simulink model "EV_TMS_MODEL"  (R2024a)
settings: Solver=VariableStepAuto  StartTime=0.0  StopTime=1000  RelTol=1e-3
values from neighbouring files (symbols this model uses):
  air_density = 1.225    [model_script.m]
  battery_C1_LUT = [1913.6 12447 30609 ... (first row only)    [model_script.m]
  battery_capacity_LUT = [280.081 276.25 276.392]    [model_script.m]
  battery_cell_cp = 795    [model_script.m]
  battery_cell_mass = 2.5    [model_script.m]
  battery_Em_LUT = [3.4966 3.5057 3.5148 ... (first row only)    [model_script.m]
  battery_N_cells = 20    [model_script.m]
  battery_Qe_init = 0    [model_script.m]
  battery_R0_LUT = [0.0117 0.0085 0.009 ... (first row only)    [model_script.m]
  battery_R1_LUT = [0.0109 0.0029 0.0013 ... (first row only)    [model_script.m]
  battery_SOC_LUT = [0; 0.1; 0.25; 0.5; 0.75; 0.9; 1]    [model_script.m]
  battery_T_init = -10    [model_script.m]
  battery_temperature_LUT = [-10 0 5 20 40]    [model_script.m]
  cabin_doors_conductivity = 0.2    [model_script.m]
  cabin_glass_conductivity = 1    [model_script.m]
  cabin_roof_conductivity = 0.2    [model_script.m]
  cabin_T_init = -10    [model_script.m]
  coolant_channel_D = 0.0092    [model_script.m]
  coolant_pipe_D = 0.02    [model_script.m]
  coolant_T_init = 30    [model_script.m]
  coolant_tank_volume = 5    [model_script.m]
  CoolingPower_kW = 3    [model_script.m]
  duct_W = 0.2    [model_script.m]
  evap_superheat_temp = 5    [model_script.m]
  pump_speed_max = 3000    [model_script.m]
  refrigerant_massflowrate = CoolingPower_kW/(evap_outlet_enthalpy-evap_inlet_enthalpy)    (= 0.0184049079755)    [model_script.m]
  RPM_Compressor_nominal = 1000    [model_script.m]
  RPM_CondFan = 3000    [model_script.m]
  RPM_EvapFan = 3000    [model_script.m]
  T_set = 20    [model_script.m]
  tube_D = 0.01    [model_script.m]
  VolFlowrate_CondenserFan = condenser_air_massflowrate/air_density    (= 0.408163265306)    [model_script.m]
  VolFlowRate_CoolantRadiatorFan = 0.5    [model_script.m]
  VolFlowRate_EvapFan = evap_air_massflowrate/air_density    (= 0.487359122754)    [model_script.m]
undefined symbols (not defined in the file or in its folder): bulb, inlet
libraries: fl_lib x238, nesl_utility x75, SimscapeFluids_lib x25, LiBatteryElements_lib x16, simulink_extras x9, slpidlib x3, autolibshared x1, SignalEditorBlockLib x1
(part 2 of 7)

== system EV_TMS_MODEL/S4 ==
  Absolute Reference (2P) : fl_lib/Two-Phase Fluid/Elements/Absolute Reference (2P)
  PS-Simulink Converter : nesl_utility/PS-Simulink Converter  PhysicalDomain=network_engine_domain  SubClassName=ps_output  LeftPortType=input  RightPortType=output  PseudoPeriodic=off  Frequencies=[]  VectorFormat=inherit  Unit=kJ/kg  AffineConversion=off
  PS-Simulink Converter1 : nesl_utility/PS-Simulink Converter  PhysicalDomain=network_engine_domain  SubClassName=ps_output  LeftPortType=input  RightPortType=output  PseudoPeriodic=off  Frequencies=[]  VectorFormat=inherit  Unit=MPa  AffineConversion=off
  Pressure & Internal Energy Sensor (2P) : fl_lib/Two-Phase Fluid/Sensors/Pressure, Temperature & Internal Energy Sensor (2P)  reference=foundation.enum.MeasurementReference.difference  pressure=true  pressure_spec=foundation.enum.PressureMeasementSpec.Absolute  temperature=false  internal_energy=true
      settings: InternalSimscapePortConfiguration="{\"Bottom\":[{\"id\":\"U\",\"label\":\"U\",\"type\":\"output\"}],\"Left\":[{\"id\":\"A\",\"label\":\"A\",\"type\":\"foundation.two_phase_fluid.two_phase_fluid\"}],\"Right\":[{\"id\":\"B\",\"label\":\"B\",\"type\":\"foundation.two_phase_fluid.two_phase_fluid\"},{\"id\":\"P\",\"label\":\"P\",\"type\":\"output\"}],\"Top\":[]}"
  Saturation Properties Sensor (2P) : fl_lib/Two-Phase Fluid/Sensors/Saturation Properties Sensor (2P)  temperature_measure=true  pressure_measure=simscape.enum.onoff.off  pressure_check=simscape.enum.assert.action.error  energy_measure=foundation.enum.EnergyMeasurement.SaturatedEnthalpy  density_measure=foundation.enum.DensityMeasurement.Off
      settings: InternalSimscapePortConfiguration="{\"Bottom\":[],\"Left\":[{\"id\":\"A\",\"label\":\"A\",\"type\":\"foundation.two_phase_fluid.two_phase_fluid\"}],\"Right\":[{\"id\":\"T_sat_liq\",\"label\":\"TL\",\"type\":\"output\"},{\"id\":\"T_sat_vap\",\"label\":\"TV\",\"type\":\"output\"}],\"Top\":[{\"id\":\"h_sat_liq\",\"label\":\"HL\",\"type\":\"output\"},{\"id\":\"h_sat_vap\",\"label\":\"HV\",\"type\":\"output\"}]}"
  Thermodynamic Properties Sensor (2P) : fl_lib/Two-Phase Fluid/Sensors/Thermodynamic Properties Sensor (2P)  temperature=true  enthalpy=true  density=false  specific_volume=true  entropy=true
      settings: InternalSimscapePortConfiguration="{\"Bottom\":[{\"id\":\"V\",\"label\":\"v\",\"type\":\"output\"},{\"id\":\"S\",\"label\":\"s\",\"type\":\"output\"}],\"Left\":[{\"id\":\"A\",\"label\":\"A\",\"type\":\"foundation.two_phase_fluid.two_phase_fluid\"}],\"Right\":[{\"id\":\"T\",\"label\":\"T\",\"type\":\"output\"},{\"id\":\"H\",\"label\":\"h\",\"type\":\"output\"}],\"Top\":[]}"
  A : PMIOPort  Side=Left
  tag scope: h4=global, p4=global
  wires:
  PS-Simulink Converter/1 -> [h4]
  PS-Simulink Converter1/1 -> [p4]
  connections:
  Pressure & Internal Energy Sensor (2P)/LConn1 -- Saturation Properties Sensor (2P)/LConn1 -- Thermodynamic Properties Sensor (2P)/LConn1 -- A/RConn1
  Absolute Reference (2P)/LConn1 -- Pressure & Internal Energy Sensor (2P)/RConn1
  PS-Simulink Converter/LConn1 -- Thermodynamic Properties Sensor (2P)/RConn2
  PS-Simulink Converter1/LConn1 -- Pressure & Internal Energy Sensor (2P)/RConn2

== system EV_TMS_MODEL/S5 ==
  Absolute Reference (2P) : fl_lib/Two-Phase Fluid/Elements/Absolute Reference (2P)
  PS-Simulink Converter : nesl_utility/PS-Simulink Converter  PhysicalDomain=network_engine_domain  SubClassName=ps_output  LeftPortType=input  RightPortType=output  PseudoPeriodic=off  Frequencies=[]  VectorFormat=inherit  Unit=kJ/kg  AffineConversion=off
  PS-Simulink Converter1 : nesl_utility/PS-Simulink Converter  PhysicalDomain=network_engine_domain  SubClassName=ps_output  LeftPortType=input  RightPortType=output  PseudoPeriodic=off  Frequencies=[]  VectorFormat=inherit  Unit=MPa  AffineConversion=off
  Pressure & Internal Energy Sensor (2P) : fl_lib/Two-Phase Fluid/Sensors/Pressure, Temperature & Internal Energy Sensor (2P)  reference=foundation.enum.MeasurementReference.difference  pressure=true  pressure_spec=foundation.enum.PressureMeasementSpec.Absolute  temperature=false  internal_energy=true
      settings: InternalSimscapePortConfiguration="{\"Bottom\":[{\"id\":\"U\",\"label\":\"U\",\"type\":\"output\"}],\"Left\":[{\"id\":\"A\",\"label\":\"A\",\"type\":\"foundation.two_phase_fluid.two_phase_fluid\"}],\"Right\":[{\"id\":\"B\",\"label\":\"B\",\"type\":\"foundation.two_phase_fluid.two_phase_fluid\"},{\"id\":\"P\",\"label\":\"P\",\"type\":\"output\"}],\"Top\":[]}"
  Saturation Properties Sensor (2P) : fl_lib/Two-Phase Fluid/Sensors/Saturation Properties Sensor (2P)  temperature_measure=true  pressure_measure=simscape.enum.onoff.off  pressure_check=simscape.enum.assert.action.error  energy_measure=foundation.enum.EnergyMeasurement.SaturatedEnthalpy  density_measure=foundation.enum.DensityMeasurement.Off
      settings: InternalSimscapePortConfiguration="{\"Bottom\":[],\"Left\":[{\"id\":\"A\",\"label\":\"A\",\"type\":\"foundation.two_phase_fluid.two_phase_fluid\"}],\"Right\":[{\"id\":\"T_sat_liq\",\"label\":\"TL\",\"type\":\"output\"},{\"id\":\"T_sat_vap\",\"label\":\"TV\",\"type\":\"output\"}],\"Top\":[{\"id\":\"h_sat_liq\",\"label\":\"HL\",\"type\":\"output\"},{\"id\":\"h_sat_vap\",\"label\":\"HV\",\"type\":\"output\"}]}"
  Thermodynamic Properties Sensor (2P) : fl_lib/Two-Phase Fluid/Sensors/Thermodynamic Properties Sensor (2P)  temperature=true  enthalpy=true  density=false  specific_volume=true  entropy=true
      settings: InternalSimscapePortConfiguration="{\"Bottom\":[{\"id\":\"V\",\"label\":\"v\",\"type\":\"output\"},{\"id\":\"S\",\"label\":\"s\",\"type\":\"output\"}],\"Left\":[{\"id\":\"A\",\"label\":\"A\",\"type\":\"foundation.two_phase_fluid.two_phase_fluid\"}],\"Right\":[{\"id\":\"T\",\"label\":\"T\",\"type\":\"output\"},{\"id\":\"H\",\"label\":\"h\",\"type\":\"output\"}],\"Top\":[]}"
  A : PMIOPort  Side=Left
  tag scope: h5=global, p5=global
  wires:
  PS-Simulink Converter/1 -> [h5]
  PS-Simulink Converter1/1 -> [p5]
  connections:
  Pressure & Internal Energy Sensor (2P)/LConn1 -- Saturation Properties Sensor (2P)/LConn1 -- Thermodynamic Properties Sensor (2P)/LConn1 -- A/RConn1
  Absolute Reference (2P)/LConn1 -- Pressure & Internal Energy Sensor (2P)/RConn1
  PS-Simulink Converter/LConn1 -- Thermodynamic Properties Sensor (2P)/RConn2
  PS-Simulink Converter1/LConn1 -- Pressure & Internal Energy Sensor (2P)/RConn2

== system EV_TMS_MODEL/Subsystem ==
  Drive Cycle Source : autolibshared/Drive Cycle Source  cycleVar=UDDS  fileVar=cycleFTP75.mat  tfinal="1369  seconds"  cycleRepeat=off  outAccPort=off  outGearPort=off  gearList=No gear data  t_wot1=5  xdot_woto=0  xdot_wot1=30  t_wot2=20  xdot_wot2=0  t_wotend=30  srcUnit=m/s  outUnit=m/s  srcAccUnit=m/s/s  outAccUnit=m/s^2  dt=0  aMode=2  faultOption=off  velBnd=2  velBndUnit=mph  inUnit=m/s  timeBnd=1  failOption=off  stopSim=off  maxFaultCnt=10  maxFaultTime=2  maxTotFaultTime=15  traceOption=off  dtTrace=1  traceWindow=10  lastDCname=UDDS  lastOutUnit=mph  lastDT=0  lastTB=1  lastSB=2  forceCalcBound=off
      settings: LibrarySourceBlock=vdynlib/Vehicle Scenarios/Drive Cycle and Maneuvers/Drive Cycle Source
  Goto : Goto  Commented=on  GotoTag=I_battery  TagVisibility=global
  Goto1 : Goto  Commented=on  GotoTag=Q_inverter  TagVisibility=global
  Goto11 : Goto  Commented=on  GotoTag=Q_charger  TagVisibility=global
  Goto3 : Goto  Commented=on  GotoTag=Q_motor  TagVisibility=global
  Goto7 : Goto  Commented=on  GotoTag=v_vehicle  TagVisibility=global
  Power Demand : Subsystem  Commented=on
  Power Demand1 : Subsystem
  Signal Editor : SignalEditorBlockLib/Signal Editor  Commented=on  FileName=EVBatteryCoolingSystem.mat  ActiveScenario=FTP_75_Drive_Cycle  ActiveSignal=Speed  IsBus=off  OutputBusObjectStr=Bus: BusObject  SampleTime=0  Interpolate=off  ZeroCross=off  OutputAfterFinalValue=Setting to zero  Unit=inherit  PreserveSignalName=on  ApplySigPropsToAllScenarios=on  ApplySigPropsToAllSignals=off
  tag scope: I_battery=global, Q_charger=global, Q_inverter=global, Q_motor=global, v_vehicle=global
  wires:
  Power Demand/4(Q_charger) -> Goto11/1
  Power Demand/2(Q_inverter) -> Goto1/1
  Power Demand/1(I_battery) -> Goto/1
  Power Demand/3(Q_motor) -> Goto3/1
  Signal Editor/1 -> Power Demand/1(speed), Goto7/1
  Signal Editor/2 -> Power Demand/2(In2)
  Power Demand1/2(Q_inverter) -> [Q_inverter]
  Power Demand1/3(Q_motor) -> [Q_motor]
  Power Demand1/1(I_battery) -> [I_battery]
  Power Demand1/4(Q_charger) -> [Q_charger]
  Drive Cycle Source/1 -> [v_vehicle], Power Demand1/1(speed)

== system EV_TMS_MODEL/Subsystem1 ==
  Sum : Sum  Inputs=|+++++
  Out1 : Outport
  wires:
  [Q_chiller] -> Sum/3  "ChillerHeat"
  [Q_coolant_radiator] -> Sum/5  "CoolantRadiatorHeat"
  [Q_cond] -> Sum/1  "CondenserHeat"
  Sum/1 -> Out1/1
  [Q_cabin] -> Sum/4  "CabinHeatExchangeToExterior"
  [Q_evap] -> Sum/2  "EvaporatorHeat"

== system EV_TMS_MODEL/Subsystem2 ==
  Sum : Sum  Inputs=|+++++
  Out1 : Outport
  wires:
  Sum/1 -> Out1/1
  [Pwr_CoolantPump] -> Sum/4  "Pwr_CoolantPump"
  [Pwr_CoolantRadiatorFan] -> Sum/5  "Pwr_CoolantRadiatorFan"
  [Pwr_Compressor] -> Sum/1  "Pwr_Compressor"
  [Pwr_CondenserFan] -> Sum/2  "Pwr_CondenserFan"
  [Pwr_BlowerFan] -> Sum/3  "Pwr_BlowerFan"

== system EV_TMS_MODEL/TXV1 ==
  note: The bulb of the TXV contains a temperature-sensitive material (such as a refrigerant) that expands or contracts based on the temperature it is exposed to. This expansion or contraction of the bulb material controls the opening and closing of the TXV valve, regulating the flow of refrigerant into the evaporator coil. The bulb temperature is typically measured at the outlet of the evaporator coil. The bulb of the TXV is attached to the suction line of the refrigeration system at the outlet of the evaporator, the line which is connected to the compressor. This placement allows the bulb to sense the temperature of the refrigerant vapor leaving the evaporator.
      | By measuring the temperature at the outlet of the evaporator, the TXV can maintain a consistent superheat level, ensuring optimal evaporator performance and preventing issues such as flooding or starving of the evaporator coil. The superheat level is the difference between the measured bulb temperature and the refrigerant saturation temperature at the evaporator outlet.
  Simscape Bus : SimscapeBus  HierarchyStrings=bulb;inlet
  Thermostatic Expansion Valve : SimscapeFluids_lib/Two-Phase Fluid/Valves & Orifices/Flow Control Valves/Thermostatic Expansion Valve (2P)  valve_parameterization=fluids.two_phase_fluid.valves_orifices.flow_control_valves.enum.ThermostaticExpansionValveParameterization.Nominal  capacity_spec=fluids.two_phase_fluid.valves_orifices.flow_control_valves.enum.ThermostaticExpansionValveCapacitySpec.MassFlowRate  Q_nominal=0.5*CoolingPower_kW kW  Q_max=0.5*CoolingPower_kW* 1.5 kW  mdot_nominal=refrigerant_massflowrate kg/s  mdot_max=1.5*refrigerant_massflowrate kg/s  pressure_spec=fluids.two_phase_fluid.valves_orifices.flow_control_valves.enum.ThermostaticExpansionValvePressureSpec.SaturationTemperature  p_cond_nominal=1.5 MPa  p_evap_nominal=0.5 MPa  T_cond_nominal=nominal_condens_temp degC  T_evap_nominal=nominal_evap_temp degC  delta_T_sub=condenser_subcooling_temp deltaK  delta_T_nominal=evap_superheat_temp deltaK  delta_T_static=0.5*evap_superheat_temp deltaK  mop=fluids.two_phase_fluid.valves_orifices.flow_control_valves.enum.ThermostaticExpansionValveMOP.Off  p_mop=0.5 MPa  T_mop=288.15 K  T_evap_out_TLU1=0 : 10 : 40 degC  p_bulb_TLU1=0.3 : 0.1 : 0.7 MPa  lift_TLU2=0 : 0.15 : 0.6 mm  p_evap_TLU2=0.3 : -0.05 : 0.1 MPa  lift_TLU3=0 : 0.15 : 0.6 mm  mdot_TLU3=0 : 0.015 : 0.06 kg/s  p_cond_ref=2 MPa  p_evap_ref=0.2 MPa  T_evap_out_ref=0 degC  delta_T_sub_ref=5 deltaK  pressure_equalization=fluids.two_phase_fluid.valves_orifices.flow_control_valves.enum.ThermostaticExpansionValveEqualization.External  bulb_dynamics=simscape.enum.onoff.off  tau_bulb=20 s  leakage_fraction=1e-6  smoothing_factor=0.5  B_lam=0.999  tau_x=0.1 s  area=pi*tube_D^2/4 m^2
      settings: InternalSimscapePortConfiguration="{\"Bottom\":[],\"Left\":[{\"id\":\"A\",\"label\":\"A\",\"type\":\"foundation.two_phase_fluid.two_phase_fluid\"}],\"Right\":[{\"id\":\"B\",\"label\":\"B\",\"type\":\"foundation.two_phase_fluid.two_phase_fluid\"}],\"Top\":[{\"id\":\"S\",\"label\":\"S\",\"type\":\"foundation.two_phase_fluid.two_phase_fluid\"},{\"id\":\"E\",\"label\":\"E\",\"type\":\"foundation.two_phase_fluid.two_phase_fluid\"}]}"
  B : PMIOPort  Side=Left
  A : PMIOPort  Port=2  Side=Right
  connections:
  B/RConn1 -- Simscape Bus/RConn1
  Thermostatic Expansion Valve/RConn1 -- Simscape Bus/LConn2
  Simscape Bus/LConn1 -- Thermostatic Expansion Valve/LConn2 -- Thermostatic Expansion Valve/LConn3
  Thermostatic Expansion Valve/LConn1 -- A/RConn1

== system EV_TMS_MODEL/TXV2 ==
  note: The bulb of the TXV contains a temperature-sensitive material (such as a refrigerant) that expands or contracts based on the temperature it is exposed to. This expansion or contraction of the bulb material controls the opening and closing of the TXV valve, regulating the flow of refrigerant into the evaporator coil. The bulb temperature is typically measured at the outlet of the evaporator coil. The bulb of the TXV is attached to the suction line of the refrigeration system at the outlet of the evaporator, the line which is connected to the compressor. This placement allows the bulb to sense the temperature of the refrigerant vapor leaving the evaporator.
      | By measuring the temperature at the outlet of the evaporator, the TXV can maintain a consistent superheat level, ensuring optimal evaporator performance and preventing issues such as flooding or starving of the evaporator coil. The superheat level is the difference between the measured bulb temperature and the refrigerant saturation temperature at the evaporator outlet.
  Chiller Expansion Valve : SimscapeFluids_lib/Two-Phase Fluid/Valves & Orifices/Flow Control Valves/Thermostatic Expansion Valve (2P)  valve_parameterization=fluids.two_phase_fluid.valves_orifices.flow_control_valves.enum.ThermostaticExpansionValveParameterization.Nominal  capacity_spec=fluids.two_phase_fluid.valves_orifices.flow_control_valves.enum.ThermostaticExpansionValveCapacitySpec.MassFlowRate  Q_nominal=CoolingPower_kW kW  Q_max=CoolingPower_kW* 1.5 kW  mdot_nominal=refrigerant_massflowrate kg/s  mdot_max=1.5*refrigerant_massflowrate kg/s  pressure_spec=fluids.two_phase_fluid.valves_orifices.flow_control_valves.enum.ThermostaticExpansionValvePressureSpec.SaturationTemperature  p_cond_nominal=1.5 MPa  p_evap_nominal=0.3 MPa  T_cond_nominal=nominal_condens_temp degC  T_evap_nominal=nominal_evap_temp degC  delta_T_sub=condenser_subcooling_temp deltaK  delta_T_nominal=evap_superheat_temp deltaK  delta_T_static=0.5*evap_superheat_temp deltaK  mop=fluids.two_phase_fluid.valves_orifices.flow_control_valves.enum.ThermostaticExpansionValveMOP.Off  p_mop=0.5 MPa  T_mop=288.15 K  T_evap_out_TLU1=0 : 10 : 40 degC  p_bulb_TLU1=0.3 : 0.1 : 0.7 MPa  lift_TLU2=0 : 0.15 : 0.6 mm  p_evap_TLU2=0.3 : -0.05 : 0.1 MPa  lift_TLU3=0 : 0.15 : 0.6 mm  mdot_TLU3=[1e-7, 0.015 : 0.015 : 0.06] kg/s  p_cond_ref=2 MPa  p_evap_ref=0.3 MPa  T_evap_out_ref=0 degC  delta_T_sub_ref=5 deltaK  pressure_equalization=fluids.two_phase_fluid.valves_orifices.flow_control_valves.enum.ThermostaticExpansionValveEqualization.External  bulb_dynamics=false  tau_bulb=20 s  leakage_fraction=1e-6  smoothing_factor=0.5  B_lam=0.999  tau_x=1 s  area=pi*tube_D^2/4 m^2
      settings: InternalSimscapePortConfiguration="{\"Bottom\":[],\"Left\":[{\"id\":\"A\",\"label\":\"A\",\"type\":\"foundation.two_phase_fluid.two_phase_fluid\"}],\"Right\":[{\"id\":\"B\",\"label\":\"B\",\"type\":\"foundation.two_phase_fluid.two_phase_fluid\"}],\"Top\":[{\"id\":\"S\",\"label\":\"S\",\"type\":\"foundation.two_phase_fluid.two_phase_fluid\"},{\"id\":\"E\",\"label\":\"E\",\"type\":\"foundation.two_phase_fluid.two_phase_fluid\"}]}"
  Simscape Bus : SimscapeBus  HierarchyStrings=bulb;inlet
  B : PMIOPort  Side=Left
  A : PMIOPort  Port=2  Side=Right
  connections:
  Simscape Bus/RConn1 -- B/RConn1
  Simscape Bus/LConn1 -- Chiller Expansion Valve/LConn2 -- Chiller Expansion Valve/LConn3
  Simscape Bus/LConn2 -- Chiller Expansion Valve/RConn1
  A/RConn1 -- Chiller Expansion Valve/LConn1

== system EV_TMS_MODEL/Cabin/Cabin ==
  Cabin and Occupants Model : Subsystem  Tag=PublishSubsystem
      settings: PortSchema="{\"entries\":[{\"content\":{\"sides\":[{\"content\":{},\"type\":\"ConnectorPlacement.EquallySpacedRectSide\",\"uuid\":\"e1f7673a-ae09-4e38-a748-d03f3a89f634\"},{\"content\":{\"connectorIds\":[\"RConn1\"],\"side\":\"RIGHT\"},\"type\":\"ConnectorPlacement.EquallySpacedRectSide\",\"uuid\":\"e2c59df4-5a81-4f6b-ab06-631ef800c0b1\"},{\"content\":{\"connectorIds\":[\"LConn1\"],\"side\":\"TOP\"},\"type\":\"ConnectorPlacement.EquallySpacedRectSide\",\"uuid\":\"19dd88a8-04e0-4296-a227-9de66059cdf8\"}]},\"type\":\"ConnectorPlacement.EquallySpacedConnector\",\"uuid\":\"cfca4f7e-9c0e-462b-910e-b09b0fceba6e\"}],\"packageUris\":[\"http://schema.mathworks.com/mf0/Connector/R2020b\"],\"version\":\"1.0\"}"
      settings: AttributesFormatString=|
      | Length= %<coolingBox_L>
      | Width= %<coolingBox_W>
      | Height= %<coolingBox_H>
      | Initial Temp= %<T_cabin_init_degC>
  Evaporator A : PMIOPort  Side=Left
  Evaporator B : PMIOPort  Port=2  Side=Left
  connections:
  Evaporator B/RConn1 -- Cabin and Occupants Model/LConn1
  Evaporator A/RConn1 -- Cabin and Occupants Model/RConn1

== system EV_TMS_MODEL/Chiller/Chiller ==
  note: Heat exchanger (system-level model) that lets the refrigerant absorb heat from the coolant.This way the coolant (water glycol) from the battery is cooled and heats the refrigerant (R410a)
  note: This is a model of a chiller that uses two-phase refrigeration circuit to cool a thermal liquid network. The thermal liquid network uses a water-based coolant fluid and the model can be expanded to model cooling of a BEV or HEV battery, DC/DC converter, inverter, electric motors, etc.
  Chiller (System-Level) : SimscapeFluids_lib/Heat Exchangers/Two-Phase Fluid - Thermal Liquid/System-Level Condenser Evaporator (2P-TL)  flow_arrangement=fluids.heat_exchangers.enum.SystemLevelFlowArrangement2PTL.Cross  wall_thermal_mass=false  mass_wall=1 kg  cp_wall=490 J/(K*kg)  nominal_init_wall=true  T_wall_init=293.15 K  area_A1=pi*tube_D^2/4 m^2  area_B1=pi*tube_D^2/4 m^2  area_A2=pi*tube_D^2/4 m^2  area_B2=pi*tube_D^2/4 m^2  operating_condition_2P=fluids.heat_exchangers.enum.SystemLevelOperatingCondition2PTL.Evaporator  mdot_nominal_2P=0.5*refrigerant_massflowrate kg/s  delta_p_nominal_2P=0.01 MPa  pressure_spec_cond_2P=fluids.heat_exchangers.enum.SystemLevelPressureSpecCondenser2P.InletPressure  pressure_spec_evap_2P=fluids.heat_exchangers.enum.SystemLevelPressureSpecEvaporator2P.EvaporatingTemperature  p_in_nominal_2P=1 MPa  T_cond_nominal_2P=313.15 K  T_evap_nominal_2P=nominal_evap_temp degC  inlet_spec_2P=fluids.heat_exchangers.enum.SystemLevelInletSpec2P.Temperature  T_in_nominal_2P=-10 degC  h_in_nominal_2P=evap_inlet_enthalpy kJ/kg  x_in_nominal_2P=1  capacity_spec_2P=fluids.heat_exchangers.enum.SystemLevelCapacitySpec.HeatTransfer  Q_nominal=0.1 kW  outlet_spec_cond_2P=fluids.heat_exchangers.enum.SystemLevelOutletSpecCondenser2P.Enthalpy  outlet_spec_evap_2P=fluids.heat_exchangers.enum.SystemLevelOutletSpecEvaporator2P.Superheating  delta_T_sub_nominal_2P=5 deltaK  delta_T_sup_nominal_2P=evap_superheat_temp deltaK  h_out_nominal_2P=250 kJ/kg  x_out_nominal_2P=0  volume_2P=0.001 m^3  nominal_init_2P=false  energy_spec_2P=foundation.enum.energy_spec.temperature  p_init_2P=evap_inlet_p MPa  T_init_2P=9 degC  x_init_2P=0.5  alpha_init_2P=0.5  h_init_2P=evap_inlet_enthalpy kJ/kg  u_init_2P=1500 kJ/kg  mdot_nominal_TL=pump_nominal_massflowrate kg/s  delta_p_nominal_TL=0.01 MPa  p_in_nominal_TL=coolant_p_init MPa  T_in_nominal_TL=coolant_T_init degC  volume_TL=0.001 m^3  nominal_init_TL=true  p_init_TL=0.101325 MPa  T_init_TL=293.15 K  a_liq_2P=0.023  a_mix_2P=0.005  a_vap_2P=0.023  b_2P=0.8  c_2P=0.33  a_TL=0.023  b_TL=0.8  c_TL=0.33
      settings: InternalSimscapePortConfiguration="{\"Bottom\":[],\"Left\":[{\"id\":\"A1\",\"label\":\"A1\",\"type\":\"foundation.two_phase_fluid.two_phase_fluid\"},{\"id\":\"B1\",\"label\":\"B1\",\"type\":\"foundation.two_phase_fluid.two_phase_fluid\"}],\"Right\":[{\"id\":\"A2\",\"label\":\"A2\",\"type\":\"foundation.thermal_liquid.thermal_liquid\"},{\"id\":\"B2\",\"label\":\"B2\",\"type\":\"foundation.thermal_liquid.thermal_liquid\"}],\"Top\":[{\"id\":\"Q1\",\"label\":\"Q1\",\"type\":\"output\"},{\"id\":\"Q2\",\"label\":\"Q2\",\"type\":\"output\"}]}"
  PS-Simulink Converter1 : nesl_utility/PS-Simulink Converter  PhysicalDomain=network_engine_domain  SubClassName=ps_output  LeftPortType=input  RightPortType=output  PseudoPeriodic=off  Frequencies=[]  VectorFormat=inherit  Unit=kW  AffineConversion=off
  Simscape Bus : SimscapeBus  HierarchyStrings=bulb;inlet
  To Compressor : PMIOPort  Side=Left
  C : PMIOPort  Port=2  Side=Left
  D : PMIOPort  Port=3  Side=Left
  To TXV : PMIOPort  Port=4  Side=Right
  Heat flow rate [kW] : Outport
  wires:
  PS-Simulink Converter1/1 -> Heat flow rate [kW]/1
  connections:
  To TXV/RConn1 -- Simscape Bus/RConn1
  Simscape Bus/LConn1 -- Chiller (System-Level)/LConn2 -- To Compressor/RConn1
  Simscape Bus/LConn2 -- Chiller (System-Level)/LConn1
  Chiller (System-Level)/RConn1 -- C/RConn1
  Chiller (System-Level)/RConn2 -- D/RConn1
  PS-Simulink Converter1/LConn1 -- Chiller (System-Level)/LConn3

== system EV_TMS_MODEL/Compressor/Compressor ==
  Compressor On/Off : Inport
  Compressor : Subsystem  Variant=on  VariantControlMode=label  LabelModeActiveChoice=Compressor_detailed
  Evap Outlet : PMIOPort  Side=Left
  Condenser Inlet : PMIOPort  Port=2  Side=Right
  Power [kW] : Outport
  wires:
  Compressor On/Off/1 -> Compressor/1(Compressor On/Off)
  Compressor/1(Power [kW]) -> Power [kW]/1
  connections:
  Evap Outlet/RConn1 -- Compressor/LConn1
  Condenser Inlet/RConn1 -- Compressor/RConn1

== system EV_TMS_MODEL/Condenser and Fan/Condenser and Fan ==
  Fan On/Off : Inport
  Condenser (System-Level) : SimscapeFluids_lib/Heat Exchangers/Two-Phase Fluid - Moist Air/System-Level Condenser Evaporator (2P-MA)  flow_arrangement=fluids.heat_exchangers.enum.SystemLevelFlowArrangement2PMA.Cross  wall_thermal_mass=simscape.enum.onoff.off  mass_wall=1 kg  cp_wall=490 J/(K*kg)  nominal_init_wall=true  T_wall_init=293.15 K  area_A1=pi*tube_D^2/4 m^2  area_B1=pi*tube_D^2/4 m^2  area_A2=duct_W^2 m^2  area_B2=duct_W^2 m^2  operating_condition_2P=fluids.heat_exchangers.enum.SystemLevelOperatingCondition2PMA.Condenser  mdot_nominal_2P=refrigerant_massflowrate kg/s  delta_p_nominal_2P=0.01 MPa  pressure_spec_cond_2P=fluids.heat_exchangers.enum.SystemLevelPressureSpecCondenser2P.CondensingTemperature  pressure_spec_evap_2P=fluids.heat_exchangers.enum.SystemLevelPressureSpecEvaporator2P.InletPressure  p_in_nominal_2P=1 MPa  T_cond_nominal_2P=nominal_condens_temp degC  T_evap_nominal_2P=243.15 K  inlet_spec_2P=fluids.heat_exchangers.enum.SystemLevelInletSpec2P.Enthalpy  T_in_nominal_2P=condenser_inlet_temp degC  h_in_nominal_2P=460 kJ/kg  x_in_nominal_2P=1  capacity_spec_2P=fluids.heat_exchangers.enum.SystemLevelCapacitySpec.OutletCondition  Q_nominal=0.01 kW  outlet_spec_cond_2P=fluids.heat_exchangers.enum.SystemLevelOutletSpecCondenser2P.Subcooling  outlet_spec_evap_2P=fluids.heat_exchangers.enum.SystemLevelOutletSpecEvaporator2P.Enthalpy  delta_T_sub_nominal_2P=condenser_subcooling_temp deltaK  delta_T_sup_nominal_2P=5 deltaK  h_out_nominal_2P=condenser_inlet_p kJ/kg  x_out_nominal_2P=0  volume_2P=0.001 m^3  nominal_init_2P=true  energy_spec_2P=foundation.enum.energy_spec.enthalpy  p_init_2P=condenser_inlet_p MPa  T_init_2P=refrig_T_init degC  x_init_2P=0.5  alpha_init_2P=0.5  h_init_2P=condenser_inlet_enthalpy kJ/kg  u_init_2P=1500 kJ/kg  mdot_nominal_MA=evap_air_massflowrate kg/s  delta_p_nominal_MA=200 Pa  p_in_nominal_MA=0.101325 MPa  T_in_nominal_MA=T_set degC  inlet_moisture_spec_MA=foundation.enum.moisture_spec.relative_humidity  RH_in_nominal_MA=0.5  x_w_in_nominal_MA=0.01  y_w_in_nominal_MA=0.01  HR_in_nominal_MA=0.01  Tw_in_nominal_MA=287 K  inlet_trace_gas_spec_MA=foundation.enum.trace_gas_spec.mole_fraction  x_g_in_nominal_MA=0.001  y_g_in_nominal_MA=0  volume_MA=0.15 m^3  nominal_init_MA=true  p_init_MA=moist_air_p_init MPa  T_init_MA=moist_air_T_init degC  moisture_spec_MA=foundation.enum.moisture_spec.relative_humidity  RH_init_MA=moist_air_RH_init  x_w_init_MA=0.01  y_w_init_MA=0.01  HR_init_MA=0.01  Tw_init_MA=287 K  trace_gas_spec_MA=foundation.enum.trace_gas_spec.mass_fraction  x_g_init_MA=0.001  y_g_init_MA=0.001  RH_ws_MA=1  a_liq_2P=0.023  a_mix_2P=0.005  a_vap_2P=0.023  b_2P=0.8  c_2P=0.33  a_MA=0.023  b_MA=0.8  c_MA=0.33
      settings: InternalSimscapePortConfiguration="{\"Bottom\":[],\"Left\":[{\"id\":\"A1\",\"label\":\"A1\",\"type\":\"foundation.two_phase_fluid.two_phase_fluid\"},{\"id\":\"B1\",\"label\":\"B1\",\"type\":\"foundation.two_phase_fluid.two_phase_fluid\"}],\"Right\":[{\"id\":\"A2\",\"label\":\"A2\",\"type\":\"foundation.moist_air.moist_air\"},{\"id\":\"B2\",\"label\":\"B2\",\"type\":\"foundation.moist_air.moist_air\"}],\"Top\":[{\"id\":\"Q1\",\"label\":\"Q1\",\"type\":\"output\"},{\"id\":\"Q2\",\"label\":\"Q2\",\"type\":\"output\"},{\"id\":\"W\",\"label\":\"W\",\"type\":\"output\"}]}"
  Fan : Subsystem  Variant=on  VariantControlMode=label  LabelModeActiveChoice=Fan_simple
  PS-Simulink Converter : nesl_utility/PS-Simulink Converter  PhysicalDomain=network_engine_domain  SubClassName=ps_output  LeftPortType=input  RightPortType=output  PseudoPeriodic=off  Frequencies=[]  VectorFormat=inherit  Unit=kW  AffineConversion=off
  Pipe pressure drop : fl_lib/Two-Phase Fluid/Elements/Flow Resistance (2P)  delta_p_nominal=100 Pa  mdot_nominal=refrigerant_massflowrate kg/s  v_nominal=0 m^3/kg  area=pi*tube_D^2/4 m^2  laminar_fraction=1e-3
      settings: InternalSimscapePortConfiguration="{\"Bottom\":[],\"Left\":[{\"id\":\"A\",\"label\":\"A\",\"type\":\"foundation.two_phase_fluid.two_phase_fluid\"}],\"Right\":[{\"id\":\"B\",\"label\":\"B\",\"type\":\"foundation.two_phase_fluid.two_phase_fluid\"}],\"Top\":[]}"
  Air Inlet : PMIOPort  Side=Left
  Air Outlet : PMIOPort  Port=2  Side=Left
  CoolSide_Condenser : PMIOPort  Port=3  Side=Right
  WarmSide_Condenser (from Compressor) : PMIOPort  Port=4  Side=Right
  Heat Power [kW] : Outport
  Fan Power [kW] : Outport  Port=2
  wires:
  Fan On/Off/1 -> Fan/1(Fan On/Off)
  Fan/1(Power [kW]) -> Fan Power [kW]/1
  PS-Simulink Converter/1 -> Heat Power [kW]/1
  connections:
  Air Outlet/RConn1 -- Condenser (System-Level)/RConn2
  Air Inlet/RConn1 -- Fan/RConn1
  Condenser (System-Level)/LConn2 -- CoolSide_Condenser/RConn1
  WarmSide_Condenser (from Compressor)/RConn1 -- Pipe pressure drop/LConn1
  PS-Simulink Converter/LConn1 -- Condenser (System-Level)/LConn4
  Pipe pressure drop/RConn1 -- Condenser (System-Level)/LConn1
  Fan/RConn2 -- Condenser (System-Level)/RConn1

== system EV_TMS_MODEL/Control/Cabin Air Control ==
  note: if the outside temperature is higher then the setpoint temperature turn off the PTC
  T_cabin : Inport
  T_setpoint : Inport  Port=2
  T_env : Inport  Port=3
  T_ptc : Inport  Port=4
  Constant : Constant  Value=0
  PID Controller : slpidlib/PID Controller  Controller=PI  Form=Ideal  TimeDomain=Continuous-time  UseExternalTs=off  SampleTime=-1  IntegratorMethod=Forward Euler  FilterMethod=Forward Euler  ControllerParametersSource=internal  P=1/50  I=1/150  UseKiTs=off  D=0  UseExternalDerivativeSource=off  N=100  UseFilter=on  TunerSelectOption=Transfer Function Based (PID Tuner App)  InitialConditionSource=internal  InitialConditionForIntegrator=0  InitialConditionForFilter=0  DifferentiatorICPrevScaledInput=0  ExternalReset=none  TrackingMode=off  Kt=1  LimitOutput=on  SatLimitsSource=internal  UpperSaturationLimit=1  LowerSaturationLimit=0  LinearizeAsGain=on  AntiWindupMode=back-calculation  Kb=1  LimitIntegrator=off  UpperIntegratorSaturationLimit=inf  LowerIntegratorSaturationLimit=-inf  POutMin=[]  POutMax=[]  IOutMin=[]  IOutMax=[]  DOutMin=[]  DOutMax=[]  NOutMin=[]  NOutMax=[]  SumOutMin=[]  SumOutMax=[]  SaturationOutMin=[]  SaturationOutMax=[]  PParamMin=[]  PParamMax=[]  IParamMin=[]  IParamMax=[]  DParamMin=[]  DParamMax=[]  NParamMin=[]  NParamMax=[]  KbParamMin=[]  KbParamMax=[]  KtParamMin=[]  KtParamMax=[]  KbOutMin=[]  KbOutMax=[]  KtOutMin=[]  KtOutMax=[]  IntegratorOutMin=[]  IntegratorOutMax=[]  FilterOutMin=[]  FilterOutMax=[]  SumI1OutMin=[]  SumI1OutMax=[]  SumI2OutMin=[]  SumI2OutMax=[]  SumI3OutMin=[]  SumI3OutMax=[]  SumI4OutMin=[]  SumI4OutMax=[]  SumDOutMin=[]  SumDOutMax=[]  DifferentiatorOutMin=[]  DifferentiatorOutMax=[]  FilterDiffOutCoefMin=[]  FilterDiffOutCoefMax=[]  ReciprocalOutMin=[]  ReciprocalOutMax=[]  SumDenOutMin=[]  SumDenOutMax=[]  SumNumOutMin=[]  SumNumOutMax=[]  DivideOutMin=[]  DivideOutMax=[]  UdiffTsProdOutMin=[]  UdiffTsProdOutMax=[]  NTsProdOutMin=[]  NTsProdOutMax=[]  UintegralTsProdOutMin=[]  UintegralTsProdOutMax=[]  UngainTsProdOutMin=[]  UngainTsProdOutMax=[]  ClampingZeroOutDataTypeStr=Inherit: Inherit via back propagation  ClampingZeroOutMin=[]  ClampingZeroOutMax=[]  FilterDenConstantOutDataTypeStr=Inherit: Inherit via back propagation  FilterDenConstantOutMin=[]  FilterDenConstantOutMax=[]  PCopyOutDataTypeStr=Inherit: Inherit via back propagation  PCopyOutMin=[]  PCopyOutMax=[]  NCopyOutDataTypeStr=Inherit: Inherit via back propagation  NCopyOutMin=[]  NCopyOutMax=[]  IntegratorContinuousStateAttributes=''  IntegratorStateMustResolveToSignalObject=off  IntegratorRTWStateStorageClass=Auto  FilterContinuousStateAttributes=''  FilterStateMustResolveToSignalObject=off  FilterRTWStateStorageClass=Auto  ParallelPVariant=Passthrough  IdealPVariant=InternalParameters  IVariant=InternalParameters  DVariant=Disabled  IntegratorVariant=Continuous  SatVariant=Enabled  AWVariant=BackCalculation  PCopyVariant=Disabled  TRVariant=Disabled  FdbkBlocksVariant=Forward  IdealPFdbkVariant=Disabled  SatFdbkVariant=Disabled  DerivativeFilterVariant=Disabled  NVariant=Disabled  NCopyVariant=Disabled_SignalSpec  FilterICVariant=Disabled  IntegratorICVariant=InternalICs  ExternalResetVariant=Disabled  TRSumVariant=Passthrough  SumFdbkVariant=Disabled  SumVariant=Sum_PI  TsampFilterVariant=InternalTs  TsampNgainVariant=Passthrough  TsampIntegralVariant=Disabled_SignalSpec  ExternalSaturationOutDataTypeStr=Inherit: Same as second input  DerivativeSourceVariant=Disabled
  Product : Product
  Relay : Relay  OnSwitchValue=45  OffSwitchValue=35  OnOutputValue=0  OffOutputValue=1  ZeroCross=off
  Sign : Signum
  Sum : Sum  Inputs=-+|
  Sum1 : Sum  Inputs=-+|
  Switch : Switch  SaturateOnIntegerOverflow=off  InputSameDT=off
  cmd_blower : Outport
  cmd_ptc : Outport  Port=2
  wires:
  T_setpoint/1 -> Sum1/1, Sum/1
  Sum1/1 -> Switch/2, Sign/1
  Product/1 -> PID Controller/1
  PID Controller/1 -> cmd_blower/1
  T_env/1 -> Sum1/2
  Sum/1 -> Product/1
  Sign/1 -> Product/2
  Constant/1 -> Switch/1
  Switch/1 -> cmd_ptc/1
  Relay/1 -> Switch/3
  T_ptc/1 -> Relay/1
  T_cabin/1 -> Sum/2

== system EV_TMS_MODEL/Control/Coolant Loop Control ==
  T_env : Inport
  T_coolant_battery_in : Inport  Port=2
  T_motor : Inport  Port=3
  T_battery : Inport  Port=4
  Battery Heater : Subsystem
  Battery Pump : Subsystem
  Motor Pump : Subsystem
  cmd_heater : Outport
  cmd_motor_pump : Outport  Port=2
  cmd_battery_pump : Outport  Port=3
  wires:
  Motor Pump/1(cmd_motor_pump) -> Battery Pump/1(cmd_motor_pump), cmd_motor_pump/1
  T_env/1 -> Battery Heater/1(T_env)
  T_coolant_battery_in/1 -> Battery Heater/2(T_coolant_battery_in)
  T_motor/1 -> Motor Pump/1(T_motor)
  Battery Heater/1(cmd_heater) -> cmd_heater/1
  Battery Pump/1(cmd_battery_pump) -> cmd_battery_pump/1
  T_battery/1 -> Battery Pump/2(T_battery)

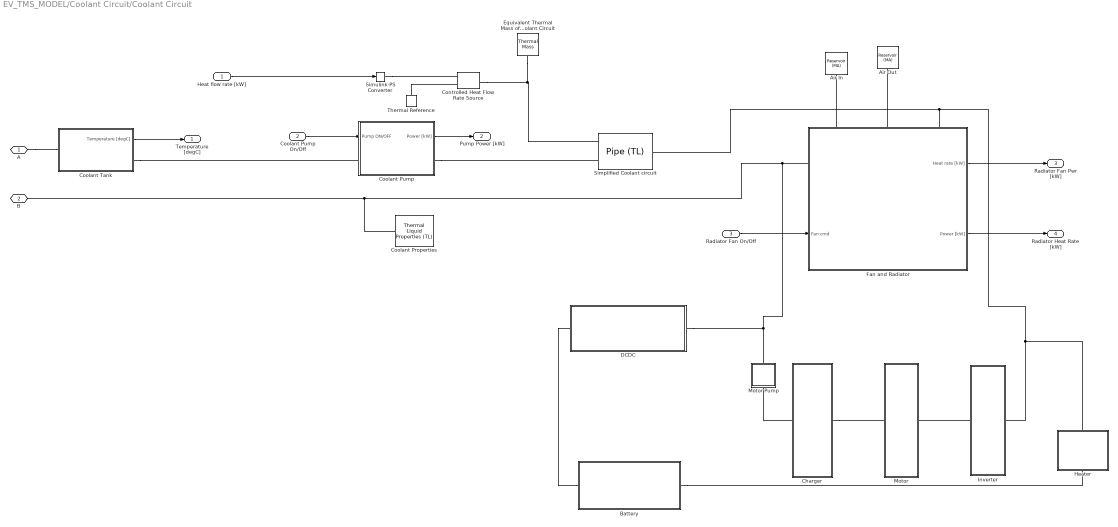
== system EV_TMS_MODEL/Coolant Circuit/Coolant Circuit ==
  Heat flow rate [kW] : Inport  Unit=kW
  Coolant Pump On/Off : Inport  Port=2
  Radiator Fan On/Off : Inport  Port=3
  Air In : fl_lib/Moist Air/Elements/Reservoir (MA)  pressure_spec=foundation.enum.pressure_spec.specified  reservoir_pressure=0.101325 MPa  temperature_spec=foundation.enum.temperature_spec.specified  reservoir_temperature=T_env degC  moisture_spec=foundation.enum.moisture_spec.relative_humidity  reservoir_RH=0.5  reservoir_x_w=0.01  reservoir_y_w=0.01  reservoir_HR=0.01  reservoir_Tw=287 K  trace_gas_spec=foundation.enum.trace_gas_spec.mole_fraction  reservoir_x_g=0.001  reservoir_y_g=0  RH_ws=1  area_A=duct_W^2 m^2
      settings: AttributesFormatString=temperature= %<reservoir_temperature>
  Air Out : fl_lib/Moist Air/Elements/Reservoir (MA)  pressure_spec=foundation.enum.pressure_spec.specified  reservoir_pressure=0.101325 MPa  temperature_spec=foundation.enum.temperature_spec.specified  reservoir_temperature=T_env degC  moisture_spec=foundation.enum.moisture_spec.relative_humidity  reservoir_RH=0.5  reservoir_x_w=0.01  reservoir_y_w=0.01  reservoir_HR=0.01  reservoir_Tw=287 K  trace_gas_spec=foundation.enum.trace_gas_spec.mole_fraction  reservoir_x_g=0.001  reservoir_y_g=0  RH_ws=1  area_A=duct_W^2 m^2
      settings: AttributesFormatString=temperature= %<reservoir_temperature>
  Battery : Subsystem  Tag=PublishSubsystem
      mask Display: disp(get_param(gcb, 'Name'))
  Charger : Subsystem  Tag=PublishSubsystem
      mask Display: disp(get_param(gcb, 'Name'))
  Controlled Heat Flow Rate Source : fl_lib/Thermal/Thermal Sources/Controlled Heat Flow Rate Source
  Coolant Properties : SimscapeFluids_lib/Thermal Liquid/Utilities/Thermal Liquid Properties (TL)  fluid_list=fluids.thermal_liquid.utilities.enum.thermal_liquid_fluid_list.ethylene_glycol  concentration_param_EG=fluids.thermal_liquid.utilities.enum.thermal_liquid_concentration.volume_fraction  concentration_param_PG=fluids.thermal_liquid.utilities.enum.thermal_liquid_concentration.volume_fraction  c_mass_SW=3.5e-3  c_mass_EG=0.1  c_mass_PG=0.1  c_mass_GL=0.1  c_vol_EG=0.5  c_vol_PG=0.1  beta_const_EG=2.1791 GPa  beta_const_PG=2.1791 GPa  beta_const_GL=2.1791 GPa  p_min_EG=0.01 MPa  p_min_PG=0.01 MPa  p_min_GL=0.01 MPa  p_max_EG=50 MPa  p_max_PG=50 MPa  p_max_GL=50 MPa  p_atm=0.101325 MPa  properties_range_check=simscape.enum.assert.action.error
  Coolant Pump : Subsystem  Tag=PublishSubsystem
      mask Display: disp(get_param(gcb, 'Name'))
  Coolant Tank : Subsystem  Tag=PublishSubsystem
      mask Display: disp(get_param(gcb, 'Name'))
  DCDC : Subsystem  Tag=PublishSubsystem
      mask Display: disp(get_param(gcb, 'Name'))
  Equivalent Thermal Mass of Coolant Circuit : fl_lib/Thermal/Thermal Elements/Thermal Mass  mass_type=foundation.enum.constant_variable.constant  mass=coolant_circuit_thermal_mass kg  sp_heat=447 J/(K*kg)  mass_min=1e-6 kg  num_ports=foundation.enum.numPorts2.one  m_specify=off  m_priority=High  m=1 kg  m_nominal_specify=off  m_nominal_value=1  m_nominal_unit=kg  T_specify=on  T_priority=High  T=coolant_T_init degC  T_nominal_specify=off  T_nominal_value=1  T_nominal_unit=K  Q_specify=off  Q_priority=None  Q=0 W  Q_nominal_specify=off  Q_nominal_value=1  Q_nominal_unit=W
  Fan and Radiator : Subsystem  Variant=on  VariantControlMode=label  LabelModeActiveChoice=Fan and Radiator
      settings: PortSchema="{\"entries\":[{\"content\":{\"sides\":[{\"content\":{\"connectorIds\":[\"LConn1\",\"In1\"]},\"type\":\"ConnectorPlacement.EquallySpacedRectSide\",\"uuid\":\"87567d80-f68c-4b64-bf6a-c400b4bb513c\"},{\"content\":{\"connectorIds\":[\"Out1\",\"Out2\"],\"side\":\"RIGHT\"},\"type\":\"ConnectorPlacement.EquallySpacedRectSide\",\"uuid\":\"13164718-8307-4ae7-9828-04a93716e2b6\"},{\"content\":{\"connectorIds\":[\"LConn2\",\"LConn3\",\"LConn4\"],\"side\":\"TOP\"},\"type\":\"ConnectorPlacement.EquallySpacedRectSide\",\"uuid\":\"880ff039-95ae-477c-b44a-94cf6e1f296b\"}]},\"type\":\"ConnectorPlacement.EquallySpacedConnector\",\"uuid\":\"bcf499af-974a-4a5a-a938-12fb51c2e8c4\"}],\"packageUris\":[\"http://schema.mathworks.com/mf0/Connector/R2020b\"],\"version\":\"1.0\"}"
      mask Display: disp(get_param(gcb, 'Name'))
  Heater : Subsystem  Tag=PublishSubsystem
      settings: PortSchema="{\"entries\":[{\"content\":{\"sides\":[{\"content\":{\"connectorIds\":[]},\"type\":\"ConnectorPlacement.EquallySpacedRectSide\",\"uuid\":\"e68f4e4f-d2a0-4f21-a3dd-a8ccea0ce87c\"},{\"content\":{\"connectorIds\":[],\"side\":\"RIGHT\"},\"type\":\"ConnectorPlacement.EquallySpacedRectSide\",\"uuid\":\"01f15736-e6d7-4b17-9e84-cef8e8356dfe\"},{\"content\":{\"connectorIds\":[\"LConn1\"],\"side\":\"TOP\"},\"type\":\"ConnectorPlacement.EquallySpacedRectSide\",\"uuid\":\"cb1790c7-7993-46e4-a971-f0b801f1d2ca\"},{\"content\":{\"connectorIds\":[\"RConn1\"],\"side\":\"BOTTOM\"},\"type\":\"ConnectorPlacement.EquallySpacedRectSide\",\"uuid\":\"c273a181-4a30-4811-b574-293af963aa70\"},{\"content\":{\"connectorIds\":[],\"side\":\"HIDDEN\"},\"type\":\"ConnectorPlacement.EquallySpacedRectSide\",\"uuid\":\"e2e3575c-3b20-453d-a897-62a34bc693b5\"}]},\"type\":\"ConnectorPlacement.EquallySpacedConnector\",\"uuid\":\"0a7b2bb7-4c38-48ec-bfc1-fef0f38ff266\"}],\"packageUris\":[\"http://schema.mathworks.com/mf0/Connector/R2020b\"],\"version\":\"1.0\"}"
      mask Display: disp(get_param(gcb, 'Name'))
  Inverter : Subsystem  Tag=PublishSubsystem
      mask Display: disp(get_param(gcb, 'Name'))
  Motor : Subsystem  Tag=PublishSubsystem
      mask Display: disp(get_param(gcb, 'Name'))
  Motor Pump : Subsystem  Tag=PublishSubsystem
      settings: PortSchema="{\"entries\":[{\"content\":{\"sides\":[{\"content\":{\"connectorIds\":[]},\"type\":\"ConnectorPlacement.EquallySpacedRectSide\",\"uuid\":\"e68f4e4f-d2a0-4f21-a3dd-a8ccea0ce87c\"},{\"content\":{\"connectorIds\":[],\"side\":\"RIGHT\"},\"type\":\"ConnectorPlacement.EquallySpacedRectSide\",\"uuid\":\"01f15736-e6d7-4b17-9e84-cef8e8356dfe\"},{\"content\":{\"connectorIds\":[\"LConn1\"],\"side\":\"TOP\"},\"type\":\"ConnectorPlacement.EquallySpacedRectSide\",\"uuid\":\"cb1790c7-7993-46e4-a971-f0b801f1d2ca\"},{\"content\":{\"connectorIds\":[\"RConn1\"],\"side\":\"BOTTOM\"},\"type\":\"ConnectorPlacement.EquallySpacedRectSide\",\"uuid\":\"8246d38e-a008-4f4a-9c4c-9e03a2298f65\"},{\"content\":{\"connectorIds\":[],\"side\":\"HIDDEN\"},\"type\":\"ConnectorPlacement.EquallySpacedRectSide\",\"uuid\":\"e2e3575c-3b20-453d-a897-62a34bc693b5\"}]},\"type\":\"ConnectorPlacement.EquallySpacedConnector\",\"uuid\":\"0a7b2bb7-4c38-48ec-bfc1-fef0f38ff266\"}],\"packageUris\":[\"http://schema.mathworks.com/mf0/Connector/R2020b\"],\"version\":\"1.0\"}"
      mask Display:
      | plot(100*cos(linspace(0, 2*pi, 500)), 100*sin(linspace(0, 2*pi, 500)))
      | patch([0 24 -24 0], [-100 -55 -55 -100]+1, [0 0 0])
  Simplified Coolant circuit : SimscapeFluids_lib/Thermal Liquid/Pipes & Fittings/Pipe (TL)  dynamic_compressibility=false  inertia=false  num_segments=1  pipe_length=coolant_circuit_length m  cross_section_geometry=fluids.thermal_liquid.pipes_fittings.enum.CrossSectionGeometry.Circular  pipe_diameter=coolant_pipe_D m  pipe_inner_diameter=0.05 m  pipe_outer_diameter=0.1 m  pipe_width=0.1 m  pipe_height=0.1 m  pipe_major_axis=0.1 m  pipe_minor_axis=0.05 m  pipe_side=0.1 m  pipe_angle=30 deg  area=0.01 m^2  Dh=0.1128 m  elevation_spec=foundation.enum.constant_variable.constant  elevation_gain=0 m  gravity_spec=foundation.enum.constant_variable.constant  g=9.81 m/s^2  pressure_loss_spec=fluids.thermal_liquid.pipes_fittings.enum.PressureLossSpec.Haaland  local_pressure_loss_spec=fluids.thermal_liquid.pipes_fittings.enum.LocalLossSpec.AggregateLength  length_add=1 m  loss_coefficient=0.1  roughness_spec=fluids.thermal_liquid.pipes_fittings.enum.RoughnessSpec.CommercialPipe  roughness=15e-6 m  Re_friction_TLU=[400, 1000, 1500, 3000, 4000, 6000, 10000, 20000, 40000, 60000, 100000, 100000000]  friction_factor_TLU=[.264, .112, .071, .0417, .0387, .0268, .025, .0232, .0226, .022, .0214, .0214]  Re_lam=2000  Re_tur=4000  shape_factor=64  mdot_nominal=[.1, 1] kg/s  p_diff_nominal=[.001, .01] MPa  mdot_threshold=1e-6 kg/s  wall_spec=fluids.thermal_liquid.pipes_fittings.enum.wall_spec.rigid  vol_expansion_spec=fluids.thermal_liquid.pipes_fittings.enum.VolumeExpansionSpec.Area  area_pressure_gain=1e-6 m^2/MPa  static_pressure_TLU=[.1, 1] MPa  area_pressure_gain_TLU=[1e-05, 1.1e-05] m^2  material_behavior_spec=fluids.thermal_liquid.pipes_fittings.enum.PipeMaterialBehavior.Linear  diameter_pressure_gain=1e-6 m/MPa  wall_thickness=0.05 m  elastic_modulus=69 GPa  stress_TLU=[276, 310] MPa  strain_TLU=[.004, .02]  stress_assert_action=simscape.enum.assert.action.none  stress_max=400 MPa  poisson_ratio=0.33  wall_time_constant=0.01 s  thermal_expansion=false  alpha_L_wall=24 um/(deltaK*m)  thermal_expansion_Tref=293.15 K  heat_transfer_spec=fluids.thermal_liquid.pipes_fittings.enum.HeatTransferSpec.Gnielinski  mdot_nominal_heat=[.1, 1] kg/s  T_in_nominal=[293.15, 293.15] K  T_out_nominal=[300, 300] K  p_in_nominal_heat=[.101325, .101325] MPa  T_wall_nominal=[303.15, 303.15] K  a_coeff=0.023  b_Re_power=0.8  c_Pr_power=0.4  Nu_lam=3.66  Re_Colburn_TLU=[100, 150, 1000]  Colburn_factor_TLU=[.019, .013, .002]  Re_Nu_TLU=[100, 150, 1000]  Pr_Nu_TLU=[1, 10]  Nu_TLU=[3.72, 4.21; 3.75, 4.44; 4.21, 7.15]  p0_vec=coolant_p_init MPa  T0_vec=coolant_T_init degC  mdot0=0.1 kg/s
  Simulink-PS Converter : nesl_utility/Simulink-PS Converter  PhysicalDomain=network_engine_domain  SubClassName=ps_input  LeftPortType=input  RightPortType=output  PseudoPeriodic=off  Frequencies=[]  NoiseDistribution=none  NoiseParameters=[]  Unit=kW  AffineConversion=off  FilteringAndDerivatives=filter  SimscapeFilterOrder=1  InputFilterTimeConstant=1  UdotUserProvided=0
  Thermal Reference : fl_lib/Thermal/Thermal Elements/Thermal Reference
  A : PMIOPort  Side=Left
  B : PMIOPort  Port=2  Side=Left
  Temperature [degC] : Outport
  Pump Power [kW] : Outport  Port=2
  Radiator Fan Pwr [kW] : Outport  Port=3
  Radiator Heat Rate [kW] : Outport  Port=4
  wires:
  Coolant Pump/1(Power [kW]) -> Pump Power [kW]/1
  Coolant Pump On/Off/1 -> Coolant Pump/1(Pump ON/OFF)
  Heat flow rate [kW]/1 -> Simulink-PS Converter/1
  Radiator Fan On/Off/1 -> Fan and Radiator/1(Fan cmd)
  Fan and Radiator/1(Heat rate [kW]) -> Radiator Fan Pwr [kW]/1
  Fan and Radiator/2(Power [kW]) -> Radiator Heat Rate [kW]/1
  Coolant Tank/1(Temperature [degC]) -> Temperature [degC]/1
  connections:
  Motor Pump/LConn1 -- DCDC/RConn1 -- Fan and Radiator/LConn1 -- Coolant Properties/RConn1 -- B/RConn1
  Coolant Pump/RConn1 -- Simplified Coolant circuit/LConn1
  Controlled Heat Flow Rate Source/LConn1 -- Equivalent Thermal Mass of Coolant Circuit/LConn1 -- Simplified Coolant circuit/LConn2
  Thermal Reference/LConn1 -- Controlled Heat Flow Rate Source/RConn2
  Simulink-PS Converter/RConn1 -- Controlled Heat Flow Rate Source/RConn1
  Fan and Radiator/LConn2 -- Air In/LConn1
  Fan and Radiator/LConn3 -- Air Out/LConn1
  DCDC/LConn1 -- Battery/LConn1
  A/RConn1 -- Coolant Tank/LConn1
  Battery/RConn1 -- Heater/RConn1
  Charger/RConn1 -- Motor/LConn1
  Inverter/LConn1 -- Motor/RConn1
  Charger/LConn1 -- Motor Pump/RConn1
  Heater/LConn1 -- Simplified Coolant circuit/RConn1 -- Fan and Radiator/LConn4 -- Inverter/RConn1
  Coolant Tank/RConn1 -- Coolant Pump/LConn1
